simulink model "model_34"  (Simulink 8.7)
settings: Solver=VariableStepAuto  StartTime=0.0  StopTime=10.0  RelTol=1e-3
values from neighbouring files (symbols this model uses):
  den_d_p = dict_d_p_tf('denominator')    [simulate_model_temperature_pressure.m]
  num_d_p = dict_d_p_tf('nominator')    [simulate_model_temperature_pressure.m]
  r = x(nb + d + 1 : end)    [get_rst_regulator.m]    (also in simulate_model_temperature_pressure.m = dict_d_r_tf('R')')
  s = tf('s')    [calculate_debit_transfer_function.m]    (also in calculate_regulator.m; get_debit_1_initial_values.m; get_debit_2_initial_values.m; get_rst_regulator.m = x(1 : nb + d))
  Ts = 0.1    [aist_script.m]    (also in get_rst_regulator.m = dict_perf_criteria('discretisation_period'))
settings Model: Creator=danba  LastModifiedBy=danba
settings DataIOCC: LimitDataPoints=off  SaveFormat=Dataset
settings DebuggingCC: UnderspecifiedInitializationDetection=Simplified  MergeDetectMultiDrivingBlocksExec=error
settings HardwareCC: ProdBitPerPointer=64  ProdLargestAtomicFloat=Float  ProdIntDivRoundTo=Zero  ProdEndianess=LittleEndian  ProdWordSize=64  ProdHWDeviceType=Intel->x86-64 (Windows64)
settings ModelReferenceCC: PropagateSignalLabelsOutOfModel=on
settings ConfigComp: CovModelRefEnable=off

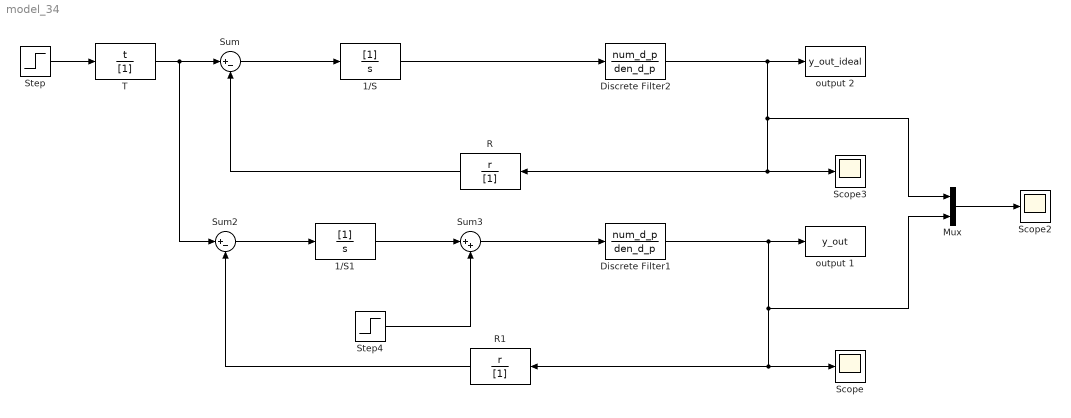
== system model_34 ==
  1/S : DiscreteFilter  Denominator=s  SampleTime=Ts
  1/S1 : DiscreteFilter  Denominator=s  SampleTime=Ts
  Discrete Filter1 : DiscreteFilter  Numerator=num_d_p  Denominator=den_d_p  SampleTime=Ts
  Discrete Filter2 : DiscreteFilter  Numerator=num_d_p  Denominator=den_d_p  SampleTime=Ts
  Mux : Mux  Inputs=2
  R : DiscreteFilter  Numerator=r  Denominator=[1]  SampleTime=Ts
  R1 : DiscreteFilter  Numerator=r  Denominator=[1]  SampleTime=Ts
  Scope : Scope
  Scope2 : Scope
  Scope3 : Scope
  Step : Step  SampleTime=0.01
  Step4 : Step  Time=3  After=0.2  SampleTime=1
  Sum : Sum  Inputs=|+-
  Sum2 : Sum  Inputs=|+-
  Sum3 : Sum  Inputs=|++
  T : DiscreteFilter  Numerator=t  Denominator=[1]  SampleTime=Ts
  output 1 : ToWorkspace  VariableName=y_out  SaveFormat=Structure With Time  SampleTime=-1
  output 2 : ToWorkspace  VariableName=y_out_ideal  SaveFormat=Structure With Time  SampleTime=-1
  wires:
  1/S/1 -> Discrete Filter2/1
  Sum/1 -> 1/S/1
  Discrete Filter2/1 -> output 2/1, R/1, Scope3/1, Mux/1
  Sum2/1 -> 1/S1/1
  Discrete Filter1/1 -> R1/1, Scope/1, Mux/2, output 1/1
  1/S1/1 -> Sum3/1
  Sum3/1 -> Discrete Filter1/1
  Step4/1 -> Sum3/2
  Mux/1 -> Scope2/1
  Step/1 -> T/1
  R/1 -> Sum/2
  T/1 -> Sum2/1, Sum/1
  R1/1 -> Sum2/2
